simulink model "SimulationModelbeforeSimX"  (R2020a)
settings: Solver=VariableStepAuto  StartTime=0.0  StopTime=SimTime  RelTol=1e-3
PreLoadFcn:
  | Simulation_parameters
InitFcn:
  | Simulation_parameters
values from neighbouring files (symbols this model uses):
  Amp_denom = 5000    [Simulation_parameters.m]
  Amp_num = 5000    [Simulation_parameters.m]
  extra = 0    [Simulation_parameters.m]
  Km = 35.6e-3    (= 0.0356)    [Simulation_parameters.m]
  Kp = 50    [Simulation_parameters.m]
  Kv = 1./(268./60*2*pi)    (= 0.0356317036773)    [Simulation_parameters.m]
  L = 1.320e-3    (= 0.00132)    [Simulation_parameters.m]
  R = 22.8    [Simulation_parameters.m]
  r2d = 180/pi    (= 57.2957795131)    [Simulation_parameters.m]
settings Model: Creator=nisch  LastModifiedBy=nisch

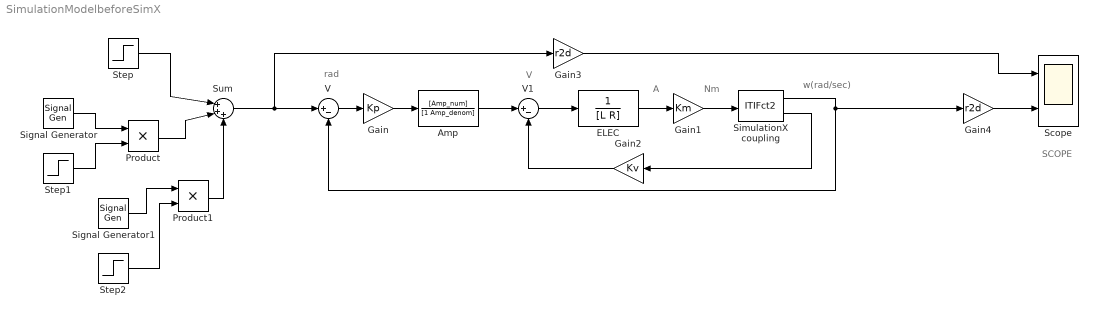
== system SimulationModelbeforeSimX ==
  note: SCOPE
  note: w(rad/sec)
  note: A
  note: V
  note: rad
  note: Nm
  Amp : TransferFcn  Numerator=[Amp_num]  Denominator=[1 Amp_denom]
  ELEC : TransferFcn  Denominator=[L R]
  Gain : Gain  Gain=Kp
  Gain1 : Gain  Gain=Km
  Gain2 : Gain  Gain=Kv
  Gain3 : Gain  Gain=r2d
  Gain4 : Gain  Gain=r2d
  Product : Product
  Product1 : Product
  Scope : Scope  NumInputPorts=2
  Signal Generator : SignalGenerator  Amplitude=pi/2*extra  Frequency=0.5
  Signal Generator1 : SignalGenerator  WaveForm=sawtooth  Amplitude=pi*extra  Frequency=2
  SimulationX coupling : S-Function  FunctionName=ITIFct2  Parameters=ip, port, ts, nIn, nOut  SFunctionDeploymentMode=off  EnableBusSupport=off  mask{ip='localhost', port=4097, ts=1e-03, nIn=1, nOut=2}
      mask prompts: ip "Address: ip"; port "Port Number: port [-]"; ts "Communication Step Size: ts [s]"; nIn "Input Vector Dimension (to SimulationX): nIn [-]"; nOut "Output Vector Dimension (from SimulationX): nOut [-]"
      mask help: Coupling Element
  Step : Step  Time=0.5  After=pi/2  SampleTime=0
  Step1 : Step  Time=0.9  Before=1  After=0  SampleTime=0
  Step2 : Step  Time=1.5  SampleTime=0
  Sum : Sum  Inputs=|+++
  V : Sum  Inputs=|+-
  V1 : Sum  Inputs=|+-
  wires:
  ELEC/1 -> Gain1/1
  V/1 -> Gain/1
  Gain1/1 -> SimulationX coupling/1
  Gain/1 -> Amp/1
  Amp/1 -> V1/1
  V1/1 -> ELEC/1
  Gain2/1 -> V1/2
  Gain3/1 -> Scope/1
  Gain4/1 -> Scope/2
  Sum/1 -> Gain3/1, V/1
  Step/1 -> Sum/1
  Signal Generator/1 -> Product/1
  Step1/1 -> Product/2
  Product/1 -> Sum/2
  Step2/1 -> Product1/2
  Signal Generator1/1 -> Product1/1
  Product1/1 -> Sum/3
  SimulationX coupling/2 -> Gain2/1
  SimulationX coupling/1 -> V/2, Gain4/1
